simulink library "uavsimBlockset_ZagiUAS"  (Simulink 8.4)
settings: Solver=ode45  StartTime=0.0  StopTime=10.0  RelTol=1e-3
undefined symbols (not defined in the file): aircraftmask_originNED_ECEF_rrm, aircraftmask_p0_NED_m, aircraftmask_phithetapsi0, aircraftmask_pqr0, aircraftmask_uvw0, Earth, fflib_degdegm2rrm, flat2lla, uavsim, WGS84
libraries: aerolibtransform2 x3, formationFlyingBlockset x3, uavsimblockset_SixDOFKinematics x2, aerolibasang x1, uavsimBlockset_StateSpaceSystem x1, uavsimBlockset_Zagi_Aerandpropulsion x1, uavsimBlockset_ElectricPropulsion x1
settings Model: Creator=mstolle  LastModifiedBy=j.bolting

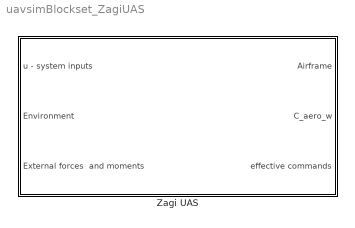
== system uavsimBlockset_ZagiUAS ==
  Zagi UAS : Subsystem  mask{mask_zagi_phithetapsi0=aircraftmask_phithetapsi0, mask_zagi_p0_ECEF_lla=fflib_degdegm2rrm(flat2lla(aircraftmask_p0_NED_m, rad2deg(aircraftmask_originNED_ECEF_rrm(1:2)), 0, aircraftmask_originNED_ECEF_rrm(3))), mask_zagi_originNED_ECEF_rrm=aircraftmask_originNED_ECEF_rrm, mask_zagi_pqr0=aircraftmask_pqr0, mask_zagi_uvw0=aircraftmask_uvw0, uavsim=uavsim}
      mask prompts: mask_zagi_phithetapsi0 "Initial euler angles [rad]"; mask_zagi_p0_ECEF_lla "Initial position ECEF [rad rad m]"; mask_zagi_originNED_ECEF_rrm "Origin NED frame, ECEF-WGS84, [rad rad m]"; mask_zagi_pqr0 "Initial body rotation rates [rad/s]"; mask_zagi_uvw0 "Initial velocity body frame [m/s]"; uavsim "Parameter set"
      mask Display: image(imread('images/zagi_slope.png'),[.3, .3, .4, .4])

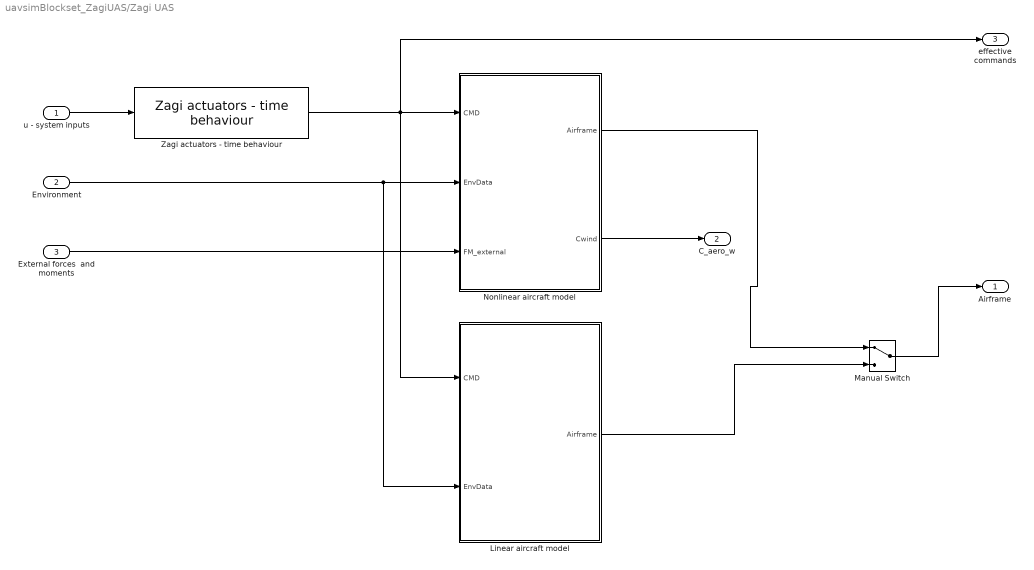
== system uavsimBlockset_ZagiUAS/Zagi UAS ==
  u - system inputs : Inport  OutDataTypeStr=Bus: CMD
  Environment : Inport  Port=2  OutDataTypeStr=Bus: Environment
  External forces  and moments : Inport  Port=3
  Linear aircraft model : Subsystem  mask{mask_ssm=uavsim.zagi.linearModels.eulers.ss_full, mask_xtrim=uavsim.zagi.x_trim, mask_utrim=uavsim.zagi.u_trim, mask_ytrim=uavsim.zagi.u_trim}
      mask prompts: mask_ssm "State space model"; mask_xtrim "x trim"; mask_utrim "u trim"; mask_ytrim "y trim"
  Manual Switch : ManualSwitch
  Nonlinear aircraft model : Subsystem
  Zagi actuators - time behaviour : formationFlyingBlockset/Zagi actuators - time behaviour
  Airframe : Outport  OutDataTypeStr=Bus: Airframe
  C_aero_w : Outport  Port=2
  effective commands : Outport  Port=3  OutDataTypeStr=Bus: CMD
  wires:
  Manual Switch/1 -> Airframe/1
  Linear aircraft model/1(Airframe) -> Manual Switch/2
  Nonlinear aircraft model/1(Airframe) -> Manual Switch/1
  Zagi actuators - time behaviour/1 -> Nonlinear aircraft model/1(CMD), effective commands/1, Linear aircraft model/1(CMD)
  External forces  and moments/1 -> Nonlinear aircraft model/3(FM_external)
  Nonlinear aircraft model/2(Cwind) -> C_aero_w/1
  u - system inputs/1 -> Zagi actuators - time behaviour/1
  Environment/1 -> Nonlinear aircraft model/2(EnvData), Linear aircraft model/2(EnvData)

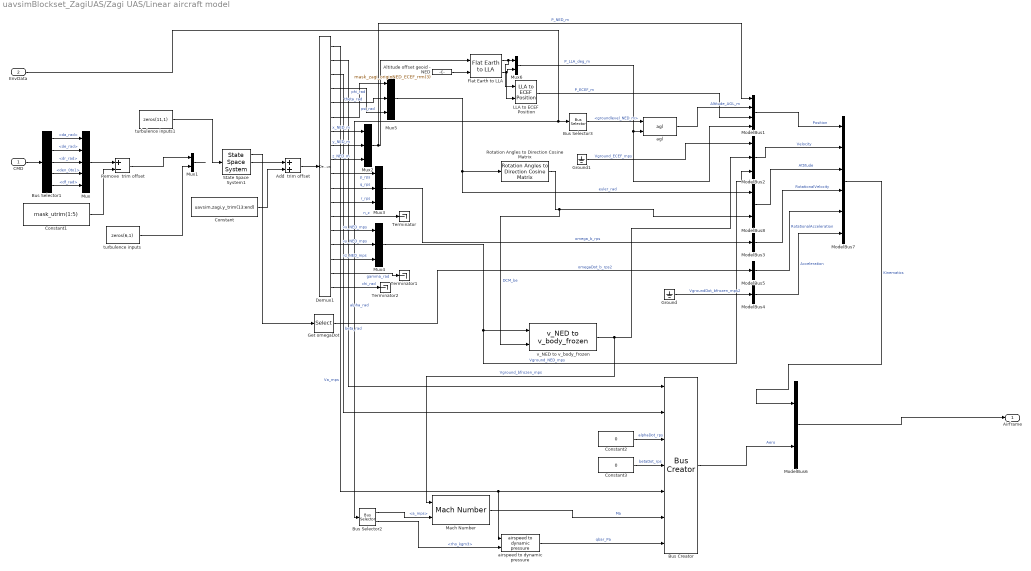
== system uavsimBlockset_ZagiUAS/Zagi UAS/Linear aircraft model ==
  CMD : Inport  OutDataTypeStr=Bus: CMD
  EnvData : Inport  Port=2
  Add  trim offset : Sum
  Altitude offset geoid - NED : Constant  Value=mask_zagi_originNED_ECEF_rrm(3)
  Bus Selector1 : BusSelector  OutputSignals=da_rad,de_rad,dr_rad,den_0to1,df_rad
  Bus Creator : BusCreator  Inputs=7
  Bus Selector2 : BusSelector  OutputSignals=a_mps,rho_kgm3
  Bus Selector3 : BusSelector  OutputSignals=groundlevel_NED_m
  Constant : Constant  Value=uavsim.zagi.y_trim(13:end)
  Constant1 : Constant  Value=mask_utrim(1:5)
  Constant2 : Constant  Value=0
  Constant3 : Constant  Value=0
  Demux1 : Demux  Outputs=18
  Flat Earth to LLA : aerolibtransform2/Flat Earth to LLA  units=Metric (MKS)  ptype=Earth (WGS84)  F=1/298.257223563  R=6378137  LL0=rad2deg(mask_zagi_originNED_ECEF_rrm(1:2))  psi=0
  Get omegaDot : Selector  InputPortWidth=12  Indices=10:12
  Ground : Ground
  Ground1 : Ground
  LLA to ECEF Position : aerolibtransform2/LLA to ECEF Position  units=Metric (MKS)  ptype=Earth (WGS84)  F=1/298.257223563  R=6378137
  Mach Number : aerolibasang/Mach Number
  ModelBus1 : BusCreator  OutDataTypeStr=Bus: Position
  ModelBus2 : BusCreator  Inputs=3  OutDataTypeStr=Bus: Velocity
  ModelBus3 : BusCreator  Inputs=1  OutDataTypeStr=Bus: RotationalVelocity
  ModelBus4 : BusCreator  Inputs=1  OutDataTypeStr=Bus: Acceleration
  ModelBus5 : BusCreator  Inputs=1  OutDataTypeStr=Bus: RotationalAcceleration
  ModelBus6 : BusCreator  Inputs=2  OutDataTypeStr=Bus: Airframe  NonVirtualBus=on
  ModelBus7 : BusCreator  Inputs=6  OutDataTypeStr=Bus: Kinematics  NonVirtualBus=on
  ModelBus8 : BusCreator  Inputs=2  OutDataTypeStr=Bus: Attitude
  Mux : Mux  Inputs=5
  Mux1 : Mux  Inputs=2
  Mux{2..5} (4 alike) : Mux  Inputs=3
  Mux6 : Mux  Inputs=2
  Remove  trim offset : Sum  Inputs=+-
  Rotation Angles to Direction Cosine Matrix : aerolibtransform2/Rotation Angles to Direction Cosine Matrix  rotationOrder=ZYX
  State Space System1 : uavsimBlockset_StateSpaceSystem/State Space System  mask_a=mask_ssm.a  mask_b=mask_ssm.b  mask_c=mask_ssm.c  mask_d=mask_ssm.d  mask_x0=mask_xtrim
  Terminator : Terminator
  Terminator1 : Terminator
  Terminator2 : Terminator
  agl : uavsimblockset_SixDOFKinematics/Aircraft kinematics/agl
  airspeed to dynamic pressure : formationFlyingBlockset/airspeed to dynamic pressure
  turbulence inputs : Constant  Value=zeros(6,1)
  turbulence inputs1 : Constant  Value=zeros(11,1)
  v_NED to v_body_frozen : formationFlyingBlockset/v_NED to v_body_frozen
  Airframe : Outport
  wires:
  turbulence inputs1/1 -> State Space System1/1
  Bus Selector2/2 -> airspeed to dynamic pressure/2  "<rho_kgm3>"
  Bus Selector2/1 -> Mach Number/2  "<a_mps>"
  State Space System1/1 -> Get omegaDot/1
  EnvData/1 -> Bus Selector2/1, Bus Selector3/1
  Flat Earth to LLA/2 -> Mux6/2, LLA to ECEF Position/2
  Flat Earth to LLA/1 -> Mux6/1, LLA to ECEF Position/1
  turbulence inputs/1 -> Mux1/2
  Mux1/1 -> ?
  Demux1/18 -> Terminator2/1  "chi_rad"
  Demux1/17 -> Terminator1/1  "gamma_rad"
  Demux1/16 -> Mux4/3  "vz_NED_mps"
  Demux1/15 -> Mux4/2  "vy_NED_mps"
  Demux1/14 -> Mux4/1  "vx_NED_mps"
  Demux1/13 -> Terminator/1  "n_z"
  Demux1/12 -> Mux3/3  "r_rps"
  Demux1/11 -> Mux3/2  "q_rps"
  Demux1/10 -> Mux3/1  "p_rps"
  Demux1/9 -> Mux2/3  "z_NED_m"
  Demux1/8 -> Mux2/2  "y_NED_m"
  Demux1/7 -> Mux2/1  "x_NED_m"
  Demux1/6 -> Mux5/1  "psi_rad"
  Demux1/5 -> Mux5/2  "theta_rad"
  Demux1/4 -> Mux5/3  "phi_rad"
  Demux1/3 -> Bus Creator/2  "beta_rad"
  Demux1/2 -> Bus Creator/1  "alpha_rad"
  Add  trim offset/1 -> Demux1/1
  Remove  trim offset/1 -> Mux1/1
  Constant1/1 -> Remove  trim offset/2
  Mux/1 -> Remove  trim offset/1
  Bus Selector1/5 -> Mux/5  "<df_rad>"
  Bus Selector1/4 -> Mux/4  "<den_0to1>"
  Bus Selector1/1 -> Mux/1  "<da_rad>"
  Bus Selector1/3 -> Mux/3  "<dr_rad>"
  Bus Selector1/2 -> Mux/2  "<de_rad>"
  CMD/1 -> Bus Selector1/1
  Constant/1 -> Add  trim offset/2
  State Space System1/2 -> Add  trim offset/1
  Mux6/1 -> agl/2, ModelBus1/4  "P_LLA_deg_m"
  Ground/1 -> ModelBus4/1  "VgroundDot_bfrozen_mps2"
  Get omegaDot/1 -> ModelBus5/1  "omegaDot_b_rps2"
  ModelBus2/1 -> ModelBus7/2  "Velocity"
  ModelBus3/1 -> ModelBus7/4  "RotationalVelocity"
  LLA to ECEF Position/1 -> ModelBus1/3  "P_ECEF_m"
  ModelBus5/1 -> ModelBus7/5  "RotationalAcceleration"
  Rotation Angles to Direction Cosine Matrix/1 -> ModelBus8/2, v_NED to v_body_frozen/2  "DCM_be"
  Mux3/1 -> ModelBus3/1  "omega_b_rps"
  ModelBus8/1 -> ModelBus7/3  "Attitude"
  agl/1 -> ModelBus1/2  "Altitude_AGL_m"
  Mux5/1 -> ModelBus8/1, Rotation Angles to Direction Cosine Matrix/1  "euler_rad"
  Mux2/1 -> Flat Earth to LLA/1, ModelBus1/1  "P_NED_m"
  ModelBus1/1 -> ModelBus7/1  "Position"
  Ground1/1 -> ModelBus2/1  "Vground_ECEF_mps"
  ModelBus4/1 -> ModelBus7/6  "Acceleration"
  v_NED to v_body_frozen/1 -> ModelBus2/2, Mach Number/1  "Vground_bfrozen_mps"
  Bus Selector3/1 -> agl/1  "<groundlevel_NED_m>"
  Altitude offset geoid - NED/1 -> Flat Earth to LLA/2
  Mux4/1 -> v_NED to v_body_frozen/1, ModelBus2/3  "Vground_NED_mps"
  Constant2/1 -> Bus Creator/3  "alphaDot_rps"
  Constant3/1 -> Bus Creator/4  "betaDot_rps"
  Demux1/1 -> Bus Creator/5, airspeed to dynamic pressure/1  "Va_mps"
  Mach Number/1 -> Bus Creator/6  "Ma"
  airspeed to dynamic pressure/1 -> Bus Creator/7  "qbar_Pa"
  Bus Creator/1 -> ModelBus6/2  "Aero"
  ModelBus6/1 -> Airframe/1
  ModelBus7/1 -> ModelBus6/1  "Kinematics"

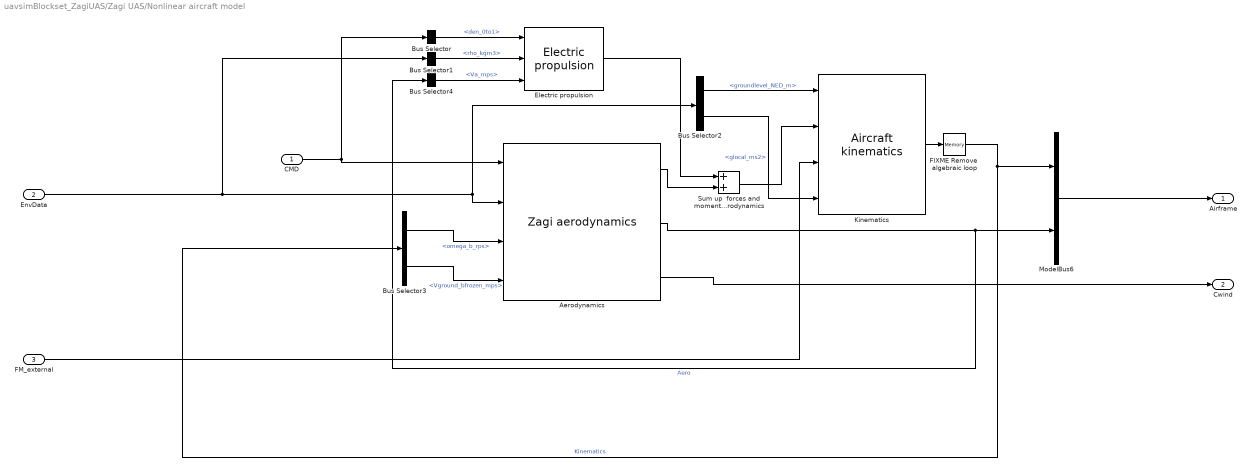
== system uavsimBlockset_ZagiUAS/Zagi UAS/Nonlinear aircraft model ==
  CMD : Inport
  EnvData : Inport  Port=2
  FM_external : Inport  Port=3
  Aerodynamics : uavsimBlockset_Zagi_Aerandpropulsion/Zagi aerodynamics
  Bus Selector : BusSelector  OutputSignals=den_0to1
  Bus Selector1 : BusSelector  OutputSignals=rho_kgm3
  Bus Selector2 : BusSelector  OutputSignals=groundlevel_NED_m,glocal_ms2
  Bus Selector3 : BusSelector  OutputSignals=RotationalVelocity.omega_b_rps,Velocity.Vground_bfrozen_mps
  Bus Selector4 : BusSelector  OutputSignals=Va_mps
  Electric propulsion : uavsimBlockset_ElectricPropulsion/Electric propulsion  mask_C_prop=uavsim.zagi.engine.C_prop  mask_S_prop=uavsim.zagi.engine.S_prop  mask_k_motor=uavsim.zagi.engine.k_motor
  FIXME Remove  algebraic loop : Memory  X0=1e-6
  Kinematics : uavsimblockset_SixDOFKinematics/Aircraft kinematics  mask_inertia=uavsim.zagi.inertiaTensor  mask_mass=uavsim.zagi.mass  mask_P0_ECEF_rrm=mask_zagi_p0_ECEF_lla  mask_originNED_ECEF_rrm=mask_zagi_originNED_ECEF_rrm  mask_uvw0=mask_zagi_uvw0  mask_phithetapsi0=mask_zagi_phithetapsi0  mask_omega0=mask_zagi_pqr0
  ModelBus6 : BusCreator  Inputs=2  OutDataTypeStr=Bus: Airframe  NonVirtualBus=on
  Sum up  forces and moments of engine and aircraft aerodynamics : Sum
  Airframe : Outport  OutDataTypeStr=Bus: Airframe
  Cwind : Outport  Port=2
  wires:
  FIXME Remove  algebraic loop/1 -> ModelBus6/1, Bus Selector3/1  "Kinematics"
  Bus Selector2/1 -> Kinematics/1  "<groundlevel_NED_m>"
  Bus Selector2/2 -> Kinematics/4  "<glocal_ms2>"
  Bus Selector3/1 -> Aerodynamics/3  "<omega_b_rps>"
  Bus Selector3/2 -> Aerodynamics/4  "<Vground_bfrozen_mps>"
  ModelBus6/1 -> Airframe/1
  Aerodynamics/2 -> Bus Selector4/1, ModelBus6/2  "Aero"
  EnvData/1 -> Bus Selector1/1, Aerodynamics/2, Bus Selector2/1
  FM_external/1 -> Kinematics/3
  Aerodynamics/3 -> Cwind/1
  Aerodynamics/1 -> Sum up  forces and moments of engine and aircraft aerodynamics/2
  Sum up  forces and moments of engine and aircraft aerodynamics/1 -> Kinematics/2
  Kinematics/1 -> FIXME Remove  algebraic loop/1
  Bus Selector4/1 -> Electric propulsion/3  "<Va_mps>"
  Bus Selector1/1 -> Electric propulsion/2  "<rho_kgm3>"
  Bus Selector/1 -> Electric propulsion/1  "<den_0to1>"
  CMD/1 -> Aerodynamics/1, Bus Selector/1
  Electric propulsion/1 -> Sum up  forces and moments of engine and aircraft aerodynamics/1
